simulink model "Exercitiul1"  (R2016a)
settings: Solver=VariableStepDiscrete  StartTime=0.0  StopTime=480  RelTol=1e-3
undefined symbols (not defined in the file): m, n
settings Model: Creator=Cristina  LastModifiedBy=Cristina

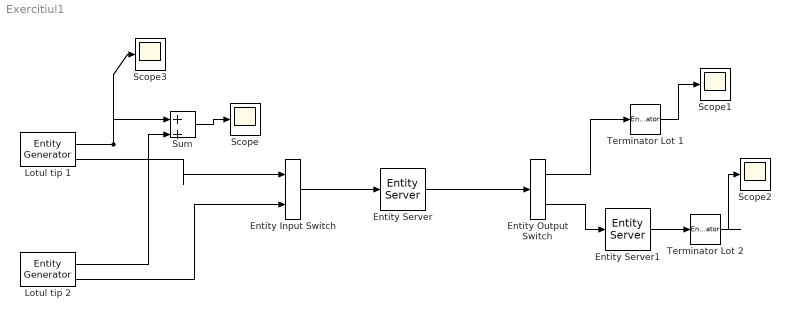
== system Exercitiul1 ==
  Entity Input Switch : EntityInputSwitch  InputPortMessageModes=m,m  OutputPortMessageModes=m
  Entity Output Switch : EntityOutputSwitch  InputPortMessageModes=m  OutputPortMessageModes=m,m  SwitchingCriterion=From attribute  SwitchAttributeName=TipLot
  Entity Server : EntityServer  InputPortMessageModes=m  OutputPortMessageModes=m  Capacity=1  ServiceTimeSource=MATLAB action  ServiceTimeAction=|
      | persistent init
      | if (isempty(init))
      |     rng(774);
      |     init = true;
      | end;
      | dt = 14 + 8 * rand;
  Entity Server1 : EntityServer  InputPortMessageModes=m  OutputPortMessageModes=m  Capacity=1  ServiceTimeSource=MATLAB action  ServiceTimeAction=|
      | persistent init
      | if (isempty(init))
      |     rng(775);
      |     init = true;
      | end;
      | dt = 8 + 4 * rand;
  Lotul tip 1 : EntityGenerator  OutputPortMessageModes=n,m  TimeSource=MATLAB action  IntergenerationTimeAction=|  AttributeName=TipLot  NumberEntitiesDeparted=on  EntityType=Structured  EntityTypeName=Entity
      | persistent init
      | if (isempty(init))
      |     rng(113);
      |     init = true;
      | end
      | dt = 25 + 20 * rand;
      settings: OutputPortMap=o0,o3
  Lotul tip 2 : EntityGenerator  OutputPortMessageModes=n,m  TimeSource=MATLAB action  IntergenerationTimeAction=|  AttributeName=TipLot  AttributeInitialValue=2  NumberEntitiesDeparted=on  EntityType=Structured  EntityTypeName=Entity
      | persistent init
      | if (isempty(init))
      |     rng(114);
      |     init = true;
      | end
      | dt = 38 + 14 * rand;
      settings: OutputPortMap=o0,o3
  Scope{,1..3} (4 alike) : Scope
  Sum : Sum  Inputs=|++
  Terminator Lot 1 : EntityTerminator  InputPortMessageModes=m  NumberEntitiesArrived=on
      settings: OutputPortMap=o0
  Terminator Lot 2 : EntityTerminator  InputPortMessageModes=m  NumberEntitiesArrived=on
      settings: OutputPortMap=o0
  wires:
  Lotul tip 1/2 -> Entity Input Switch/1
  Entity Output Switch/1 -> Terminator Lot 1/1
  Lotul tip 1/1 -> Scope3/1, Sum/1
  Lotul tip 2/1 -> Sum/2
  Sum/1 -> Scope/1
  Lotul tip 2/2 -> Entity Input Switch/2
  Entity Input Switch/1 -> Entity Server/1
  Entity Server/1 -> Entity Output Switch/1
  Entity Server1/1 -> Terminator Lot 2/1
  Entity Output Switch/2 -> Entity Server1/1
  Terminator Lot 1/1 -> Scope1/1
  Terminator Lot 2/1 -> Scope2/1
